simulink model "tx2"  (R2022a)
settings: Solver=FixedStepDiscrete  StartTime=0.0  StopTime=3.1e6  FixedStep=1  RelTol=1e-3
undefined symbols (not defined in the file or in its folder): rom_bf1, rom_bf2, rom_bf3, rom_bf4, rom_bf5, rom_bf6, rom_bf7, rom_bf8, rom_pilot_tt
libraries: hdlsllib x809, whdlutilities x460, whdlmod x104, whdledac x26, simulink x3
(part 1 of 27)
settings Model: SimulationMode=accelerator  Creator=admin  LastModifiedBy=admin
settings DataIOCC: ExternalInput=data_tt,valid_tt  LoadExternalInput=on

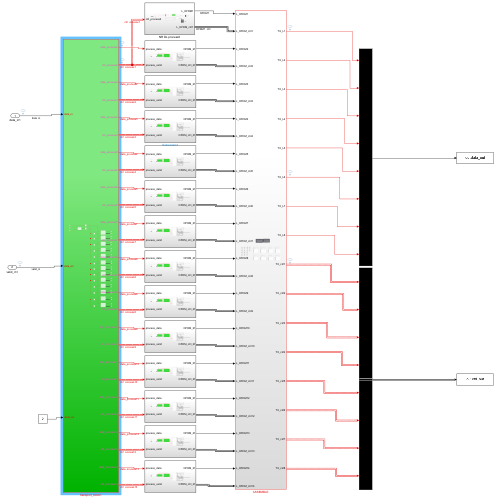
[thumbnail: Simulink's stored preview of the top-level diagram]
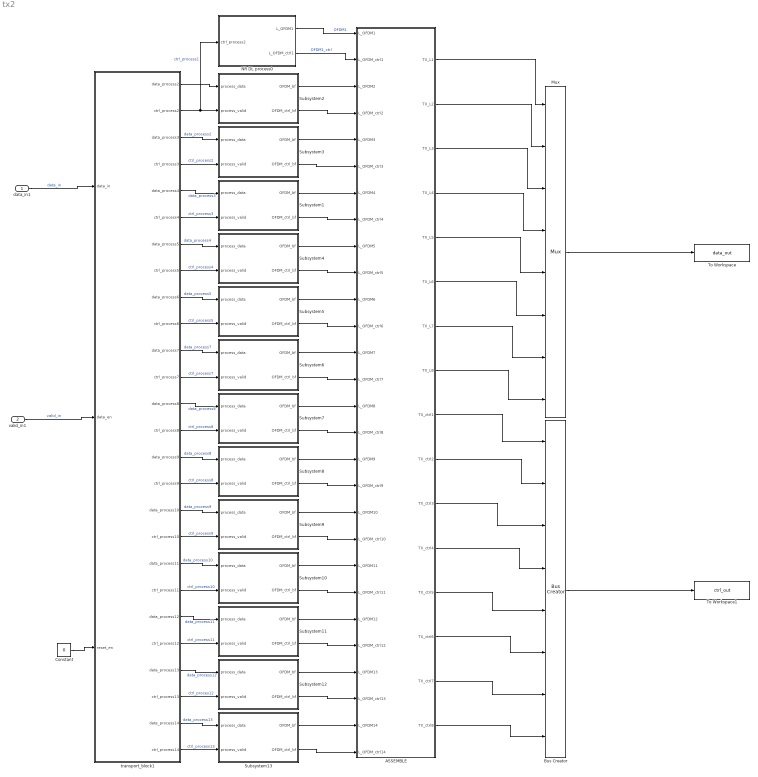
== system tx2 ==
  data_in1 : Inport  OutDataTypeStr=boolean
  valid_in1 : Inport  Port=2  OutDataTypeStr=boolean
  ASSEMBLE : Subsystem
  Bus Creator : BusCreator  Inputs=8
  Constant : Constant  Value=0  OutDataTypeStr=boolean
  Mux : Mux  Inputs=8
  NR DL process0 : Subsystem
  Subsystem1 : Subsystem
  Subsystem10 : Subsystem
  Subsystem11 : Subsystem
  Subsystem12 : Subsystem
  Subsystem13 : Subsystem
  Subsystem2 : Subsystem
  Subsystem3 : Subsystem
  Subsystem4 : Subsystem
  Subsystem5 : Subsystem
  Subsystem6 : Subsystem
  Subsystem7 : Subsystem
  Subsystem8 : Subsystem
  Subsystem9 : Subsystem
  To Workspace : ToWorkspace  VariableName=data_out  SaveFormat=Timeseries  SampleTime=-1
  To Workspace1 : ToWorkspace  VariableName=ctrl_out  SaveFormat=Timeseries  SampleTime=-1
  transport_block1 : Subsystem
  wires:
  ASSEMBLE/5(TX_L5) -> Mux/5
  transport_block1/22(ctrl_process12) -> Subsystem11/2(process_valid)  "ctrl_process11"
  Subsystem10/2(OFDM_ctrl_bf) -> ASSEMBLE/22(L_OFDM_ctrl11)
  ASSEMBLE/9(TX_ctrl1) -> Bus Creator/1
  transport_block1/25(data_process14) -> Subsystem13/1(process_data)  "data_process13"
  Subsystem11/2(OFDM_ctrl_bf) -> ASSEMBLE/24(L_OFDM_ctrl12)
  Subsystem10/1(OFDM_bf) -> ASSEMBLE/21(L_OFDM11)
  Subsystem12/2(OFDM_ctrl_bf) -> ASSEMBLE/26(L_OFDM_ctrl13)
  Subsystem9/2(OFDM_ctrl_bf) -> ASSEMBLE/20(L_OFDM_ctrl10)
  transport_block1/17(data_process10) -> Subsystem9/1(process_data)  "data_process9"
  transport_block1/20(ctrl_process11) -> Subsystem10/2(process_valid)  "ctrl_process10"
  transport_block1/8(ctrl_process5) -> Subsystem4/2(process_valid)  "ctrl_process4"
  Subsystem12/1(OFDM_bf) -> ASSEMBLE/25(L_OFDM13)
  transport_block1/14(ctrl_process8) -> Subsystem7/2(process_valid)  "ctrl_process8"
  Subsystem8/2(OFDM_ctrl_bf) -> ASSEMBLE/18(L_OFDM_ctrl9)
  Subsystem8/1(OFDM_bf) -> ASSEMBLE/17(L_OFDM9)
  transport_block1/16(ctrl_process9) -> Subsystem8/2(process_valid)  "ctrl_process8"
  Subsystem1/1(OFDM_bf) -> ASSEMBLE/7(L_OFDM4)
  Subsystem3/2(OFDM_ctrl_bf) -> ASSEMBLE/6(L_OFDM_ctrl3)
  transport_block1/4(ctrl_process3) -> Subsystem3/2(process_valid)  "ctrl_process2"
  Subsystem7/1(OFDM_bf) -> ASSEMBLE/15(L_OFDM8)
  Subsystem6/2(OFDM_ctrl_bf) -> ASSEMBLE/14(L_OFDM_ctrl7)
  transport_block1/13(data_process8) -> Subsystem7/1(process_data)  "data_process8"
  Subsystem2/2(OFDM_ctrl_bf) -> ASSEMBLE/4(L_OFDM_ctrl2)
  transport_block1/9(data_process6) -> Subsystem5/1(process_data)  "data_process5"
  transport_block1/12(ctrl_process7) -> Subsystem6/2(process_valid)  "ctrl_process7"
  Subsystem2/1(OFDM_bf) -> ASSEMBLE/3(L_OFDM2)
  Subsystem3/1(OFDM_bf) -> ASSEMBLE/5(L_OFDM3)
  ASSEMBLE/2(TX_L2) -> Mux/2
  Subsystem13/1(OFDM_bf) -> ASSEMBLE/27(L_OFDM14)
  transport_block1/10(ctrl_process6) -> Subsystem5/2(process_valid)  "ctrl_process5"
  transport_block1/6(ctrl_process4) -> Subsystem1/2(process_valid)  "ctrl_process3"
  Subsystem4/1(OFDM_bf) -> ASSEMBLE/9(L_OFDM5)
  Subsystem9/1(OFDM_bf) -> ASSEMBLE/19(L_OFDM10)
  Subsystem6/1(OFDM_bf) -> ASSEMBLE/13(L_OFDM7)
  Subsystem1/2(OFDM_ctrl_bf) -> ASSEMBLE/8(L_OFDM_ctrl4)
  transport_block1/18(ctrl_process10) -> Subsystem9/2(process_valid)  "ctrl_process9"
  ASSEMBLE/15(TX_ctrl7) -> Bus Creator/7
  Constant/1 -> transport_block1/3(reset_en)
  transport_block1/21(data_process12) -> Subsystem11/1(process_data)  "data_process11"
  transport_block1/24(ctrl_process13) -> Subsystem12/2(process_valid)  "ctrl_proces12"
  transport_block1/23(data_process13) -> Subsystem12/1(process_data)  "data_process12"
  ASSEMBLE/10(TX_ctrl2) -> Bus Creator/2
  Subsystem11/1(OFDM_bf) -> ASSEMBLE/23(L_OFDM12)
  valid_in1/1 -> transport_block1/2(data_en)  "valid_in"
  Subsystem4/2(OFDM_ctrl_bf) -> ASSEMBLE/10(L_OFDM_ctrl5)
  ASSEMBLE/1(TX_L1) -> Mux/1
  ASSEMBLE/4(TX_L4) -> Mux/4
  ASSEMBLE/12(TX_ctrl4) -> Bus Creator/4
  transport_block1/5(data_process4) -> Subsystem1/1(process_data)  "data_process3"
  NR DL process0/2(L_OFDM_ctrl1) -> ASSEMBLE/2(L_OFDM_ctrl1)  "OFDM1_ctrl"
  transport_block1/15(data_process9) -> Subsystem8/1(process_data)  "data_process8"
  ASSEMBLE/3(TX_L3) -> Mux/3
  ASSEMBLE/6(TX_L6) -> Mux/6
  ASSEMBLE/14(TX_ctrl6) -> Bus Creator/6
  ASSEMBLE/16(TX_ctrl8) -> Bus Creator/8
  transport_block1/11(data_process7) -> Subsystem6/1(process_data)  "data_process7"
  ASSEMBLE/7(TX_L7) -> Mux/7
  transport_block1/3(data_process3) -> Subsystem3/1(process_data)  "data_process2"
  NR DL process0/1(L_OFDM1) -> ASSEMBLE/1(L_OFDM1)  "OFDM1"
  transport_block1/26(ctrl_process14) -> Subsystem13/2(process_valid)  "ctrl_process13"
  ASSEMBLE/11(TX_ctrl3) -> Bus Creator/3
  data_in1/1 -> transport_block1/1(data_in)  "data_in"
  Subsystem5/2(OFDM_ctrl_bf) -> ASSEMBLE/12(L_OFDM_ctrl6)
  Subsystem7/2(OFDM_ctrl_bf) -> ASSEMBLE/16(L_OFDM_ctrl8)
  transport_block1/2(ctrl_process2) -> Subsystem2/2(process_valid), NR DL process0/1(ctrl_process2)  "ctrl_process1"
  transport_block1/19(data_process11) -> Subsystem10/1(process_data)  "data_process10"
  transport_block1/1(data_process2) -> Subsystem2/1(process_data)
  ASSEMBLE/8(TX_L8) -> Mux/8
  Subsystem5/1(OFDM_bf) -> ASSEMBLE/11(L_OFDM6)
  Subsystem13/2(OFDM_ctrl_bf) -> ASSEMBLE/28(L_OFDM_ctrl14)
  ASSEMBLE/13(TX_ctrl5) -> Bus Creator/5
  transport_block1/7(data_process5) -> Subsystem4/1(process_data)  "data_process4"
  Bus Creator/1 -> To Workspace1/1
  Mux/1 -> To Workspace/1

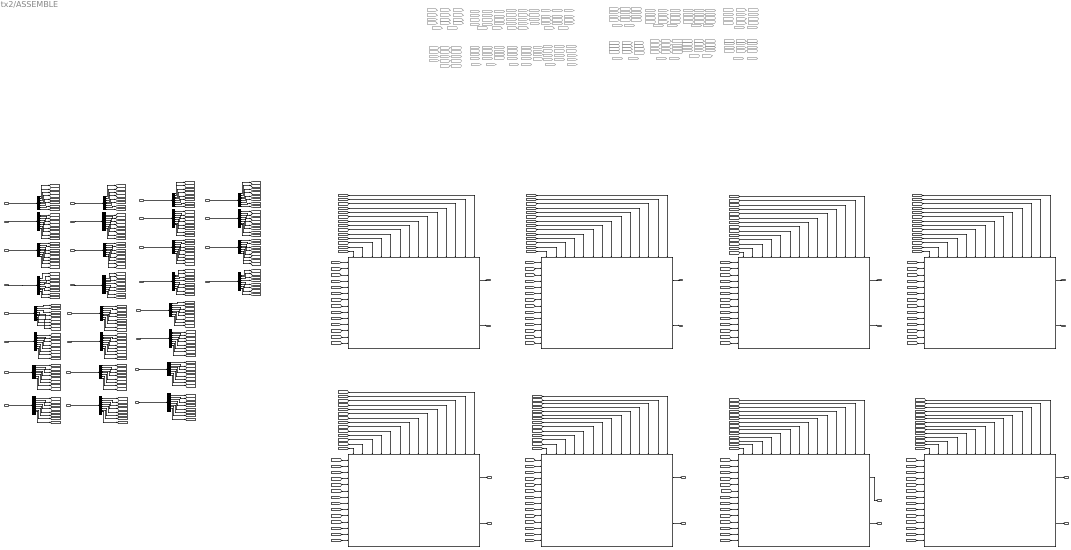
== system tx2/ASSEMBLE ==
  L_OFDM1 : Inport  PortDimensions=8
  L_OFDM_ctrl1 : Inport  Port=2  OutDataTypeStr=Bus: BUSOFDM1
  L_OFDM2 : Inport  Port=3  PortDimensions=8
  L_OFDM_ctrl2 : Inport  Port=4  OutDataTypeStr=Bus: BUSOFDM2
  L_OFDM3 : Inport  Port=5  PortDimensions=8
  L_OFDM_ctrl3 : Inport  Port=6  OutDataTypeStr=Bus: BUSOFDM3
  L_OFDM4 : Inport  Port=7  PortDimensions=8
  L_OFDM_ctrl4 : Inport  Port=8  OutDataTypeStr=Bus: BUSOFDM4
  L_OFDM5 : Inport  Port=9  PortDimensions=8
  L_OFDM_ctrl5 : Inport  Port=10  OutDataTypeStr=Bus: BUSOFDM5
  L_OFDM6 : Inport  Port=11  PortDimensions=8
  L_OFDM_ctrl6 : Inport  Port=12  OutDataTypeStr=Bus: BUSOFDM6
  L_OFDM7 : Inport  Port=13  PortDimensions=8
  L_OFDM_ctrl7 : Inport  Port=14  OutDataTypeStr=Bus: BUSOFDM7
  L_OFDM8 : Inport  Port=15  PortDimensions=8
  L_OFDM_ctrl8 : Inport  Port=16  OutDataTypeStr=Bus: BUSOFDM8
  L_OFDM9 : Inport  Port=17  PortDimensions=8
  L_OFDM_ctrl9 : Inport  Port=18  OutDataTypeStr=Bus: BUSOFDM9
  L_OFDM10 : Inport  Port=19  PortDimensions=8
  L_OFDM_ctrl10 : Inport  Port=20  OutDataTypeStr=Bus: BUSOFDM10
  L_OFDM11 : Inport  Port=21  PortDimensions=8
  L_OFDM_ctrl11 : Inport  Port=22  OutDataTypeStr=Bus: BUSOFDM11
  L_OFDM12 : Inport  Port=23  PortDimensions=8
  L_OFDM_ctrl12 : Inport  Port=24  OutDataTypeStr=Bus: BUSOFDM12
  L_OFDM13 : Inport  Port=25  PortDimensions=8
  L_OFDM_ctrl13 : Inport  Port=26  OutDataTypeStr=Bus: BUSOFDM13
  L_OFDM14 : Inport  Port=27  PortDimensions=8
  L_OFDM_ctrl14 : Inport  Port=28  OutDataTypeStr=Bus: BUSOFDM14
  Bus Selector{,2..13} (13 alike) : BusSelector  OutputSignals=L1,L2,L3,L4,L5,L6,L7,L8
  Bus Selector1 : BusSelector  OutputSignals=rom_valid (signal 1),rom_valid (signal 2),rom_valid (signal 3),rom_valid (signal 4),rom_valid (signal 5),rom_valid (signal 6),rom_valid (signal 7),rom_valid (signal 8)
  Demux{,2,4,6,8,10,12,14,16,18,24,26,28,30} (14 alike) : Demux  Outputs=8
  From : From  Commented=on  GotoTag=OFDM1_L1
  From1 : From  Commented=on  GotoTag=OFDM1_L2
  From10 : From  Commented=on  GotoTag=OFDM1_L3_C
  From100 : From  Commented=on  GotoTag=OFDM7_L5
  From101 : From  Commented=on  GotoTag=OFDM7_L6
  From102 : From  Commented=on  GotoTag=OFDM7_L7
  From103 : From  Commented=on  GotoTag=OFDM7_L8
  From104 : From  Commented=on  GotoTag=OFDM7_L1_C
  From105 : From  Commented=on  GotoTag=OFDM7_L2_C
  From106 : From  Commented=on  GotoTag=OFDM7_L3_C
  From107 : From  Commented=on  GotoTag=OFDM7_L4_C
  From108 : From  Commented=on  GotoTag=OFDM7_L5_C
  From109 : From  Commented=on  GotoTag=OFDM7_L6_C
  From11 : From  Commented=on  GotoTag=OFDM1_L4_C
  From110 : From  Commented=on  GotoTag=OFDM7_L7_C
  From111 : From  Commented=on  GotoTag=OFDM7_L8_C
  From112 : From  Commented=on  GotoTag=OFDM8_L1
  From113 : From  Commented=on  GotoTag=OFDM8_L2
  From114 : From  Commented=on  GotoTag=OFDM8_L3
  From115 : From  Commented=on  GotoTag=OFDM8_L4
  From116 : From  Commented=on  GotoTag=OFDM8_L5
  From117 : From  Commented=on  GotoTag=OFDM8_L6
  From118 : From  Commented=on  GotoTag=OFDM8_L7
  From119 : From  Commented=on  GotoTag=OFDM8_L8
  From12 : From  Commented=on  GotoTag=OFDM1_L5_C
  From120 : From  Commented=on  GotoTag=OFDM8_L1_C
  From121 : From  Commented=on  GotoTag=OFDM8_L2_C
  From122 : From  Commented=on  GotoTag=OFDM8_L3_C
  From123 : From  Commented=on  GotoTag=OFDM8_L4_C
  From124 : From  Commented=on  GotoTag=OFDM8_L5_C
  From125 : From  Commented=on  GotoTag=OFDM8_L6_C
  From126 : From  Commented=on  GotoTag=OFDM8_L7_C
  From127 : From  Commented=on  GotoTag=OFDM8_L8_C
  From128 : From  Commented=on  GotoTag=OFDM9_L1
  From129 : From  Commented=on  GotoTag=OFDM9_L2
  From13 : From  Commented=on  GotoTag=OFDM1_L6_C
  From130 : From  Commented=on  GotoTag=OFDM9_L3
  From131 : From  Commented=on  GotoTag=OFDM9_L4
  From132 : From  Commented=on  GotoTag=OFDM9_L5
  From133 : From  Commented=on  GotoTag=OFDM9_L6
  From134 : From  Commented=on  GotoTag=OFDM9_L7
  From135 : From  Commented=on  GotoTag=OFDM9_L8
  From136 : From  Commented=on  GotoTag=OFDM9_L1_C
  From137 : From  Commented=on  GotoTag=OFDM9_L2_C
  From138 : From  Commented=on  GotoTag=OFDM9_L3_C
  From139 : From  Commented=on  GotoTag=OFDM9_L4_C
  From14 : From  Commented=on  GotoTag=OFDM1_L7_C
  From140 : From  Commented=on  GotoTag=OFDM9_L5_C
  From141 : From  Commented=on  GotoTag=OFDM9_L7_C
  From142 : From  Commented=on  GotoTag=OFDM9_L6_C
  From143 : From  Commented=on  GotoTag=OFDM9_L8_C
  From144 : From  Commented=on  GotoTag=OFDM10_L1
  From145 : From  Commented=on  GotoTag=OFDM10_L2
  From146 : From  Commented=on  GotoTag=OFDM10_L3
  From147 : From  Commented=on  GotoTag=OFDM10_L4
  From148 : From  Commented=on  GotoTag=OFDM10_L5
  From149 : From  Commented=on  GotoTag=OFDM10_L6
  From15 : From  Commented=on  GotoTag=OFDM1_L8_C
  From150 : From  Commented=on  GotoTag=OFDM10_L7
  From151 : From  Commented=on  GotoTag=OFDM10_L8
  From152 : From  Commented=on  GotoTag=OFDM10_L1_C
  From153 : From  Commented=on  GotoTag=OFDM10_L2_C
  From154 : From  Commented=on  GotoTag=OFDM10_L3_C
  From155 : From  Commented=on  GotoTag=OFDM10_L4_C
  From156 : From  Commented=on  GotoTag=OFDM10_L5_C
  From157 : From  Commented=on  GotoTag=OFDM10_L6_C
  From158 : From  Commented=on  GotoTag=OFDM10_L7_C
  From159 : From  Commented=on  GotoTag=OFDM10_L8_C
  From16 : From  Commented=on  GotoTag=OFDM2_L1
  From160 : From  Commented=on  GotoTag=OFDM11_L1
  From161 : From  Commented=on  GotoTag=OFDM11_L2
  From162 : From  Commented=on  GotoTag=OFDM11_L3
  From163 : From  Commented=on  GotoTag=OFDM11_L4
  From164 : From  Commented=on  GotoTag=OFDM11_L5
  From165 : From  Commented=on  GotoTag=OFDM11_L6
  From166 : From  Commented=on  GotoTag=OFDM11_L7
  From167 : From  Commented=on  GotoTag=OFDM11_L8
  From168 : From  Commented=on  GotoTag=OFDM11_L1_C
  From169 : From  Commented=on  GotoTag=OFDM11_L2_C
  From17 : From  Commented=on  GotoTag=OFDM2_L2
  From170 : From  Commented=on  GotoTag=OFDM11_L3_C
  From171 : From  Commented=on  GotoTag=OFDM11_L4_C
  From172 : From  Commented=on  GotoTag=OFDM11_L5_C
  From173 : From  Commented=on  GotoTag=OFDM11_L6_C
  From174 : From  Commented=on  GotoTag=OFDM11_L7_C
  From175 : From  Commented=on  GotoTag=OFDM11_L8_C
  From176 : From  Commented=on  GotoTag=OFDM12_L1
  From177 : From  Commented=on  GotoTag=OFDM12_L2
  From178 : From  Commented=on  GotoTag=OFDM12_L3
  From179 : From  Commented=on  GotoTag=OFDM12_L4
  From18 : From  Commented=on  GotoTag=OFDM2_L3
  From180 : From  Commented=on  GotoTag=OFDM12_L5
  From181 : From  Commented=on  GotoTag=OFDM12_L6
  From182 : From  Commented=on  GotoTag=OFDM12_L7
  From183 : From  Commented=on  GotoTag=OFDM12_L8
  From184 : From  Commented=on  GotoTag=OFDM12_L1_C
  From185 : From  Commented=on  GotoTag=OFDM12_L2_C
  From186 : From  Commented=on  GotoTag=OFDM12_L3_C
  From187 : From  Commented=on  GotoTag=OFDM12_L4_C
  From188 : From  Commented=on  GotoTag=OFDM12_L5_C
  From189 : From  Commented=on  GotoTag=OFDM12_L6_C
  From19 : From  Commented=on  GotoTag=OFDM2_L4
  From190 : From  Commented=on  GotoTag=OFDM12_L7_C
  From191 : From  Commented=on  GotoTag=OFDM12_L8_C
  From192 : From  Commented=on  GotoTag=OFDM13_L1
  From193 : From  Commented=on  GotoTag=OFDM13_L2
  From194 : From  Commented=on  GotoTag=OFDM13_L3
  From195 : From  Commented=on  GotoTag=OFDM13_L4
  From196 : From  Commented=on  GotoTag=OFDM13_L5
  From197 : From  Commented=on  GotoTag=OFDM13_L6
  From198 : From  Commented=on  GotoTag=OFDM13_L7
  From199 : From  Commented=on  GotoTag=OFDM13_L8
  From2 : From  Commented=on  GotoTag=OFDM1_L3
  From20 : From  Commented=on  GotoTag=OFDM2_L5
  From200 : From  Commented=on  GotoTag=OFDM13_L1_C
  From201 : From  Commented=on  GotoTag=OFDM13_L2_C
  From202 : From  Commented=on  GotoTag=OFDM13_L3_C
  From203 : From  Commented=on  GotoTag=OFDM13_L4_C
  From204 : From  Commented=on  GotoTag=OFDM13_L5_C
  From205 : From  Commented=on  GotoTag=OFDM13_L6_C
  From206 : From  Commented=on  GotoTag=OFDM13_L7_C
  From207 : From  Commented=on  GotoTag=OFDM13_L8_C
  From208 : From  Commented=on  GotoTag=OFDM14_L1
  From209 : From  Commented=on  GotoTag=OFDM14_L2
  From21 : From  Commented=on  GotoTag=OFDM2_L6
  From210 : From  Commented=on  GotoTag=OFDM14_L3
  From211 : From  Commented=on  GotoTag=OFDM14_L4
  From212 : From  Commented=on  GotoTag=OFDM14_L5
  From213 : From  Commented=on  GotoTag=OFDM14_L6
  From214 : From  Commented=on  GotoTag=OFDM14_L7
  From215 : From  Commented=on  GotoTag=OFDM14_L8
  From216 : From  Commented=on  GotoTag=OFDM14_L1_C
  From217 : From  Commented=on  GotoTag=OFDM14_L2_C
  From218 : From  Commented=on  GotoTag=OFDM14_L3_C
  From219 : From  Commented=on  GotoTag=OFDM14_L4_C
  From22 : From  Commented=on  GotoTag=OFDM2_L7
  From220 : From  Commented=on  GotoTag=OFDM14_L5_C
  From221 : From  Commented=on  GotoTag=OFDM14_L6_C
  From222 : From  Commented=on  GotoTag=OFDM14_L7_C
  From223 : From  Commented=on  GotoTag=OFDM14_L8_C
  From23 : From  Commented=on  GotoTag=OFDM2_L8
  From24 : From  Commented=on  GotoTag=OFDM2_L1_C
  From25 : From  Commented=on  GotoTag=OFDM2_L2_C
  From26 : From  Commented=on  GotoTag=OFDM2_L3_C
  From27 : From  Commented=on  GotoTag=OFDM2_L4_C
  From28 : From  Commented=on  GotoTag=OFDM2_L5_C
  From29 : From  Commented=on  GotoTag=OFDM2_L6_C
  From3 : From  Commented=on  GotoTag=OFDM1_L4
  From30 : From  Commented=on  GotoTag=OFDM2_L7_C
  From31 : From  Commented=on  GotoTag=OFDM2_L8_C
  From32 : From  Commented=on  GotoTag=OFDM3_L1
  From33 : From  Commented=on  GotoTag=OFDM3_L2
  From34 : From  Commented=on  GotoTag=OFDM3_L3
  From35 : From  Commented=on  GotoTag=OFDM3_L4
  From36 : From  Commented=on  GotoTag=OFDM3_L5
  From37 : From  Commented=on  GotoTag=OFDM3_L6
  From38 : From  Commented=on  GotoTag=OFDM3_L7
  From39 : From  Commented=on  GotoTag=OFDM3_L8
  From4 : From  Commented=on  GotoTag=OFDM1_L5
  From40 : From  Commented=on  GotoTag=OFDM3_L1_C
  From41 : From  Commented=on  GotoTag=OFDM3_L2_C
  From42 : From  Commented=on  GotoTag=OFDM3_L3_C
  From43 : From  Commented=on  GotoTag=OFDM3_L4_C
  From44 : From  Commented=on  GotoTag=OFDM3_L5_C
  From45 : From  Commented=on  GotoTag=OFDM3_L6_C
  From46 : From  Commented=on  GotoTag=OFDM3_L7_C
  From47 : From  Commented=on  GotoTag=OFDM3_L8_C
  From48 : From  Commented=on  GotoTag=OFDM4_L1
  From49 : From  Commented=on  GotoTag=OFDM4_L2
  From5 : From  Commented=on  GotoTag=OFDM1_L6
  From50 : From  Commented=on  GotoTag=OFDM4_L3
  From51 : From  Commented=on  GotoTag=OFDM4_L4
  From52 : From  Commented=on  GotoTag=OFDM4_L5
  From53 : From  Commented=on  GotoTag=OFDM4_L6
  From54 : From  Commented=on  GotoTag=OFDM4_L7
  From55 : From  Commented=on  GotoTag=OFDM4_L8
  From56 : From  Commented=on  GotoTag=OFDM4_L1_C
  From57 : From  Commented=on  GotoTag=OFDM4_L2_C
  From58 : From  Commented=on  GotoTag=OFDM4_L3_C
  From59 : From  Commented=on  GotoTag=OFDM4_L4_C
  From6 : From  Commented=on  GotoTag=OFDM1_L7
  From60 : From  Commented=on  GotoTag=OFDM4_L5_C
  From61 : From  Commented=on  GotoTag=OFDM4_L6_C
  From62 : From  Commented=on  GotoTag=OFDM4_L7_C
  From63 : From  Commented=on  GotoTag=OFDM4_L8_C
  From64 : From  Commented=on  GotoTag=OFDM5_L1
  From65 : From  Commented=on  GotoTag=OFDM5_L2
  From66 : From  Commented=on  GotoTag=OFDM5_L3
  From67 : From  Commented=on  GotoTag=OFDM5_L4
  From68 : From  Commented=on  GotoTag=OFDM5_L5
  From69 : From  Commented=on  GotoTag=OFDM5_L6
  From7 : From  Commented=on  GotoTag=OFDM1_L8
  From70 : From  Commented=on  GotoTag=OFDM5_L7
  From71 : From  Commented=on  GotoTag=OFDM5_L8
  From72 : From  Commented=on  GotoTag=OFDM5_L1_C
  From73 : From  Commented=on  GotoTag=OFDM5_L2_C
  From74 : From  Commented=on  GotoTag=OFDM5_L3_C
  From75 : From  Commented=on  GotoTag=OFDM5_L4_C
  From76 : From  Commented=on  GotoTag=OFDM5_L5_C
  From77 : From  Commented=on  GotoTag=OFDM5_L6_C
  From78 : From  Commented=on  GotoTag=OFDM5_L7_C
  From79 : From  Commented=on  GotoTag=OFDM5_L8_C
  From8 : From  Commented=on  GotoTag=OFDM1_L1_C
  From80 : From  Commented=on  GotoTag=OFDM6_L1
  From81 : From  Commented=on  GotoTag=OFDM6_L2
  From82 : From  Commented=on  GotoTag=OFDM6_L3
  From83 : From  Commented=on  GotoTag=OFDM6_L4
  From84 : From  Commented=on  GotoTag=OFDM6_L5
  From85 : From  Commented=on  GotoTag=OFDM6_L6
  From86 : From  Commented=on  GotoTag=OFDM6_L7
  From87 : From  Commented=on  GotoTag=OFDM6_L8
  From88 : From  Commented=on  GotoTag=OFDM6_L1_C
  From89 : From  Commented=on  GotoTag=OFDM6_L2_C
  From9 : From  Commented=on  GotoTag=OFDM1_L2_C
  From90 : From  Commented=on  GotoTag=OFDM6_L3_C
  From91 : From  Commented=on  GotoTag=OFDM6_L4_C
  From92 : From  Commented=on  GotoTag=OFDM6_L5_C
  From93 : From  Commented=on  GotoTag=OFDM6_L6_C
  From94 : From  Commented=on  GotoTag=OFDM6_L7_C
  From95 : From  Commented=on  GotoTag=OFDM6_L8_C
  From96 : From  Commented=on  GotoTag=OFDM7_L1
  From97 : From  Commented=on  GotoTag=OFDM7_L2
  From98 : From  Commented=on  GotoTag=OFDM7_L3
  From99 : From  Commented=on  GotoTag=OFDM7_L4
  LAY1 : Subsystem
      settings: PortSchema="{\"entries\":[{\"content\":{\"sides\":[{\"content\":{\"connectorIds\":[\"In1\",\"In2\",\"In3\",\"In4\",\"In5\",\"In6\",\"In7\",\"In8\",\"In9\",\"In10\",\"In11\",\"In12\",\"In13\",\"In14\"]},\"type\":\"ConnectorPlacement.EquallySpacedRectSide\",\"uuid\":\"490598a8-c3f5-4389-b0d6-cf6a9e30693d\"},{\"content\":{\"connectorIds\":[\"Out1\",\"Out2\"],\"side\":\"RIGHT\"},\"type\":\"ConnectorPlacement.EquallySpacedRectSide\",\"uuid\":\"6437ac82-c6ba-4d32-8bfc-bd63e74c8be4\"},{\"content\":{\"connectorIds\":[\"In15\",\"In16\",\"In17\",\"In18\",\"In19\",\"In20\",\"In21\",\"In22\",\"In23\",\"In24\",\"In25\",\"In26\",\"In27\",\"In28\"],\"side\":\"TOP\"},\"type\":\"ConnectorPlacement.EquallySpacedRectSide\",\"uuid\":\"6de7b101-133c-4248-a10a-e7ae53670d39\"}]},\"type\":\"ConnectorPlacement.EquallySpacedConnector\",\"uuid\":\"6f2047fb-9444-475d-b0d6-20b25d9f763e\"}],\"packageUris\":[\"http://schema.mathworks.com/mf0/Connector/R2020b\"],\"version\":\"1.0\"}"
  LAY2 : Subsystem
      settings: PortSchema="{\"entries\":[{\"content\":{\"sides\":[{\"content\":{\"connectorIds\":[\"In1\",\"In2\",\"In3\",\"In4\",\"In5\",\"In6\",\"In7\",\"In8\",\"In9\",\"In10\",\"In11\",\"In12\",\"In13\",\"In14\"]},\"type\":\"ConnectorPlacement.EquallySpacedRectSide\",\"uuid\":\"490598a8-c3f5-4389-b0d6-cf6a9e30693d\"},{\"content\":{\"connectorIds\":[\"Out1\",\"Out2\"],\"side\":\"RIGHT\"},\"type\":\"ConnectorPlacement.EquallySpacedRectSide\",\"uuid\":\"6437ac82-c6ba-4d32-8bfc-bd63e74c8be4\"},{\"content\":{\"connectorIds\":[\"In15\",\"In16\",\"In17\",\"In18\",\"In19\",\"In20\",\"In21\",\"In22\",\"In23\",\"In24\",\"In25\",\"In26\",\"In27\",\"In28\"],\"side\":\"TOP\"},\"type\":\"ConnectorPlacement.EquallySpacedRectSide\",\"uuid\":\"6de7b101-133c-4248-a10a-e7ae53670d39\"}]},\"type\":\"ConnectorPlacement.EquallySpacedConnector\",\"uuid\":\"6f2047fb-9444-475d-b0d6-20b25d9f763e\"}],\"packageUris\":[\"http://schema.mathworks.com/mf0/Connector/R2020b\"],\"version\":\"1.0\"}"
  LAY3 : Subsystem
      settings: PortSchema="{\"entries\":[{\"content\":{\"sides\":[{\"content\":{\"connectorIds\":[\"In1\",\"In2\",\"In3\",\"In4\",\"In5\",\"In6\",\"In7\",\"In8\",\"In9\",\"In10\",\"In11\",\"In12\",\"In13\",\"In14\"]},\"type\":\"ConnectorPlacement.EquallySpacedRectSide\",\"uuid\":\"490598a8-c3f5-4389-b0d6-cf6a9e30693d\"},{\"content\":{\"connectorIds\":[\"Out1\",\"Out2\"],\"side\":\"RIGHT\"},\"type\":\"ConnectorPlacement.EquallySpacedRectSide\",\"uuid\":\"6437ac82-c6ba-4d32-8bfc-bd63e74c8be4\"},{\"content\":{\"connectorIds\":[\"In15\",\"In16\",\"In17\",\"In18\",\"In19\",\"In20\",\"In21\",\"In22\",\"In23\",\"In24\",\"In25\",\"In26\",\"In27\",\"In28\"],\"side\":\"TOP\"},\"type\":\"ConnectorPlacement.EquallySpacedRectSide\",\"uuid\":\"6de7b101-133c-4248-a10a-e7ae53670d39\"}]},\"type\":\"ConnectorPlacement.EquallySpacedConnector\",\"uuid\":\"6f2047fb-9444-475d-b0d6-20b25d9f763e\"}],\"packageUris\":[\"http://schema.mathworks.com/mf0/Connector/R2020b\"],\"version\":\"1.0\"}"
  LAY4 : Subsystem
      settings: PortSchema="{\"entries\":[{\"content\":{\"sides\":[{\"content\":{\"connectorIds\":[\"In1\",\"In2\",\"In3\",\"In4\",\"In5\",\"In6\",\"In7\",\"In8\",\"In9\",\"In10\",\"In11\",\"In12\",\"In13\",\"In14\"]},\"type\":\"ConnectorPlacement.EquallySpacedRectSide\",\"uuid\":\"490598a8-c3f5-4389-b0d6-cf6a9e30693d\"},{\"content\":{\"connectorIds\":[\"Out1\",\"Out2\"],\"side\":\"RIGHT\"},\"type\":\"ConnectorPlacement.EquallySpacedRectSide\",\"uuid\":\"6437ac82-c6ba-4d32-8bfc-bd63e74c8be4\"},{\"content\":{\"connectorIds\":[\"In15\",\"In16\",\"In17\",\"In18\",\"In19\",\"In20\",\"In21\",\"In22\",\"In23\",\"In24\",\"In25\",\"In26\",\"In27\",\"In28\"],\"side\":\"TOP\"},\"type\":\"ConnectorPlacement.EquallySpacedRectSide\",\"uuid\":\"6de7b101-133c-4248-a10a-e7ae53670d39\"}]},\"type\":\"ConnectorPlacement.EquallySpacedConnector\",\"uuid\":\"6f2047fb-9444-475d-b0d6-20b25d9f763e\"}],\"packageUris\":[\"http://schema.mathworks.com/mf0/Connector/R2020b\"],\"version\":\"1.0\"}"
  LAY5 : Subsystem
      settings: PortSchema="{\"entries\":[{\"content\":{\"sides\":[{\"content\":{\"connectorIds\":[\"In1\",\"In2\",\"In3\",\"In4\",\"In5\",\"In6\",\"In7\",\"In8\",\"In9\",\"In10\",\"In11\",\"In12\",\"In13\",\"In14\"]},\"type\":\"ConnectorPlacement.EquallySpacedRectSide\",\"uuid\":\"490598a8-c3f5-4389-b0d6-cf6a9e30693d\"},{\"content\":{\"connectorIds\":[\"Out1\",\"Out2\"],\"side\":\"RIGHT\"},\"type\":\"ConnectorPlacement.EquallySpacedRectSide\",\"uuid\":\"6437ac82-c6ba-4d32-8bfc-bd63e74c8be4\"},{\"content\":{\"connectorIds\":[\"In15\",\"In16\",\"In17\",\"In18\",\"In19\",\"In20\",\"In21\",\"In22\",\"In23\",\"In24\",\"In25\",\"In26\",\"In27\",\"In28\"],\"side\":\"TOP\"},\"type\":\"ConnectorPlacement.EquallySpacedRectSide\",\"uuid\":\"6de7b101-133c-4248-a10a-e7ae53670d39\"}]},\"type\":\"ConnectorPlacement.EquallySpacedConnector\",\"uuid\":\"6f2047fb-9444-475d-b0d6-20b25d9f763e\"}],\"packageUris\":[\"http://schema.mathworks.com/mf0/Connector/R2020b\"],\"version\":\"1.0\"}"
  LAY6 : Subsystem
      settings: PortSchema="{\"entries\":[{\"content\":{\"sides\":[{\"content\":{\"connectorIds\":[\"In1\",\"In2\",\"In3\",\"In4\",\"In5\",\"In6\",\"In7\",\"In8\",\"In9\",\"In10\",\"In11\",\"In12\",\"In13\",\"In14\"]},\"type\":\"ConnectorPlacement.EquallySpacedRectSide\",\"uuid\":\"490598a8-c3f5-4389-b0d6-cf6a9e30693d\"},{\"content\":{\"connectorIds\":[\"Out1\",\"Out2\"],\"side\":\"RIGHT\"},\"type\":\"ConnectorPlacement.EquallySpacedRectSide\",\"uuid\":\"6437ac82-c6ba-4d32-8bfc-bd63e74c8be4\"},{\"content\":{\"connectorIds\":[\"In15\",\"In16\",\"In17\",\"In18\",\"In19\",\"In20\",\"In21\",\"In22\",\"In23\",\"In24\",\"In25\",\"In26\",\"In27\",\"In28\"],\"side\":\"TOP\"},\"type\":\"ConnectorPlacement.EquallySpacedRectSide\",\"uuid\":\"6de7b101-133c-4248-a10a-e7ae53670d39\"}]},\"type\":\"ConnectorPlacement.EquallySpacedConnector\",\"uuid\":\"6f2047fb-9444-475d-b0d6-20b25d9f763e\"}],\"packageUris\":[\"http://schema.mathworks.com/mf0/Connector/R2020b\"],\"version\":\"1.0\"}"
  LAY7 : Subsystem
      settings: PortSchema="{\"entries\":[{\"content\":{\"sides\":[{\"content\":{\"connectorIds\":[\"In1\",\"In2\",\"In3\",\"In4\",\"In5\",\"In6\",\"In7\",\"In8\",\"In9\",\"In10\",\"In11\",\"In12\",\"In13\",\"In14\"]},\"type\":\"ConnectorPlacement.EquallySpacedRectSide\",\"uuid\":\"490598a8-c3f5-4389-b0d6-cf6a9e30693d\"},{\"content\":{\"connectorIds\":[\"Out1\",\"Out2\"],\"side\":\"RIGHT\"},\"type\":\"ConnectorPlacement.EquallySpacedRectSide\",\"uuid\":\"6437ac82-c6ba-4d32-8bfc-bd63e74c8be4\"},{\"content\":{\"connectorIds\":[\"In15\",\"In16\",\"In17\",\"In18\",\"In19\",\"In20\",\"In21\",\"In22\",\"In23\",\"In24\",\"In25\",\"In26\",\"In27\",\"In28\"],\"side\":\"TOP\"},\"type\":\"ConnectorPlacement.EquallySpacedRectSide\",\"uuid\":\"6de7b101-133c-4248-a10a-e7ae53670d39\"}]},\"type\":\"ConnectorPlacement.EquallySpacedConnector\",\"uuid\":\"6f2047fb-9444-475d-b0d6-20b25d9f763e\"}],\"packageUris\":[\"http://schema.mathworks.com/mf0/Connector/R2020b\"],\"version\":\"1.0\"}"
  LAY9 : Subsystem
      settings: PortSchema="{\"entries\":[{\"content\":{\"sides\":[{\"content\":{\"connectorIds\":[\"In1\",\"In2\",\"In3\",\"In4\",\"In5\",\"In6\",\"In7\",\"In8\",\"In9\",\"In10\",\"In11\",\"In12\",\"In13\",\"In14\"]},\"type\":\"ConnectorPlacement.EquallySpacedRectSide\",\"uuid\":\"490598a8-c3f5-4389-b0d6-cf6a9e30693d\"},{\"content\":{\"connectorIds\":[\"Out1\",\"Out2\"],\"side\":\"RIGHT\"},\"type\":\"ConnectorPlacement.EquallySpacedRectSide\",\"uuid\":\"6437ac82-c6ba-4d32-8bfc-bd63e74c8be4\"},{\"content\":{\"connectorIds\":[\"In15\",\"In16\",\"In17\",\"In18\",\"In19\",\"In20\",\"In21\",\"In22\",\"In23\",\"In24\",\"In25\",\"In26\",\"In27\",\"In28\"],\"side\":\"TOP\"},\"type\":\"ConnectorPlacement.EquallySpacedRectSide\",\"uuid\":\"6de7b101-133c-4248-a10a-e7ae53670d39\"}]},\"type\":\"ConnectorPlacement.EquallySpacedConnector\",\"uuid\":\"6f2047fb-9444-475d-b0d6-20b25d9f763e\"}],\"packageUris\":[\"http://schema.mathworks.com/mf0/Connector/R2020b\"],\"version\":\"1.0\"}"
  TX_L1 : Outport
      settings: SignalType=complex
  TX_L2 : Outport  Port=2
      settings: SignalType=complex
  TX_L3 : Outport  Port=3
      settings: SignalType=complex
  TX_L4 : Outport  Port=4
      settings: SignalType=complex
  TX_L5 : Outport  Port=5
      settings: SignalType=complex
  TX_L6 : Outport  Port=6
      settings: SignalType=complex
  TX_L7 : Outport  Port=7
      settings: SignalType=complex
  TX_L8 : Outport  Port=8
      settings: SignalType=complex
  TX_ctrl1 : Outport  Port=9  OutDataTypeStr=Bus: samplecontrol
  TX_ctrl2 : Outport  Port=10  OutDataTypeStr=Bus: samplecontrol
  TX_ctrl3 : Outport  Port=11  OutDataTypeStr=Bus: samplecontrol
  TX_ctrl4 : Outport  Port=12  OutDataTypeStr=Bus: samplecontrol
  TX_ctrl5 : Outport  Port=13  OutDataTypeStr=Bus: samplecontrol
  TX_ctrl6 : Outport  Port=14  OutDataTypeStr=Bus: samplecontrol
  TX_ctrl7 : Outport  Port=15  OutDataTypeStr=Bus: samplecontrol
  TX_ctrl8 : Outport  Port=16  OutDataTypeStr=Bus: samplecontrol
  wires:
  L_OFDM1/1 -> Demux/1
  L_OFDM_ctrl1/1 -> Bus Selector1/1
  L_OFDM_ctrl2/1 -> Bus Selector/1
  L_OFDM2/1 -> Demux2/1
  L_OFDM4/1 -> Demux6/1
  L_OFDM_ctrl4/1 -> Bus Selector3/1
  L_OFDM_ctrl3/1 -> Bus Selector2/1
  L_OFDM3/1 -> Demux4/1
  Demux/1 -> [OFDM1_L1]  "OFDM1"
  Demux/2 -> [OFDM1_L2]
  Demux/3 -> [OFDM1_L3]
  Demux/4 -> [OFDM1_L4]
  Demux/5 -> [OFDM1_L5]
  Demux/6 -> [OFDM1_L6]
  Demux/7 -> [OFDM1_L7]
  Demux/8 -> [OFDM1_L8]
  Bus Selector1/1 -> [OFDM1_L1_C]  "<rom_valid (signal 1)>"
  Bus Selector1/2 -> [OFDM1_L2_C]  "<rom_valid (signal 2)>"
  Bus Selector1/3 -> [OFDM1_L3_C]  "<rom_valid (signal 3)>"
  Bus Selector1/4 -> [OFDM1_L4_C]  "<rom_valid (signal 4)>"
  Bus Selector1/5 -> [OFDM1_L5_C]  "<rom_valid (signal 5)>"
  Bus Selector1/6 -> [OFDM1_L6_C]  "<rom_valid (signal 6)>"
  Bus Selector1/7 -> [OFDM1_L7_C]  "<rom_valid (signal 7)>"
  Bus Selector1/8 -> [OFDM1_L8_C]  "<rom_valid (signal 8)>"
  Demux2/1 -> [OFDM2_L1]  "OFDM2"
  Demux2/2 -> [OFDM2_L2]
  Demux2/3 -> [OFDM2_L3]
  Demux2/4 -> [OFDM2_L4]
  Demux2/5 -> [OFDM2_L5]
  Demux2/6 -> [OFDM2_L6]
  Demux2/7 -> [OFDM2_L7]
  Demux2/8 -> [OFDM2_L8]
  Bus Selector/1 -> [OFDM2_L1_C]  "<L1>"
  Bus Selector/2 -> [OFDM2_L2_C]  "<L2>"
  Bus Selector/3 -> [OFDM2_L3_C]  "<L3>"
  Bus Selector/4 -> [OFDM2_L4_C]  "<L4>"
  Bus Selector/5 -> [OFDM2_L5_C]  "<L5>"
  Bus Selector/6 -> [OFDM2_L6_C]  "<L6>"
  Bus Selector/7 -> [OFDM2_L7_C]  "<L7>"
  Bus Selector/8 -> [OFDM2_L8_C]  "<L8>"
  Demux4/1 -> [OFDM3_L1]  "OFDM3"
  Demux4/2 -> [OFDM3_L2]
  Demux4/3 -> [OFDM3_L3]
  Demux4/4 -> [OFDM3_L4]
  Demux4/5 -> [OFDM3_L5]
  Demux4/6 -> [OFDM3_L6]
  Demux4/7 -> [OFDM3_L7]
  Demux4/8 -> [OFDM3_L8]
  Bus Selector2/1 -> [OFDM3_L1_C]  "<L1>"
  Bus Selector2/2 -> [OFDM3_L2_C]  "<L2>"
  Bus Selector2/3 -> [OFDM3_L3_C]  "<L3>"
  Bus Selector2/4 -> [OFDM3_L4_C]  "<L4>"
  Bus Selector2/5 -> [OFDM3_L5_C]  "<L5>"
  Bus Selector2/6 -> [OFDM3_L6_C]  "<L6>"
  Bus Selector2/7 -> [OFDM3_L7_C]  "<L7>"
  Bus Selector2/8 -> [OFDM3_L8_C]  "<L8>"
  Demux6/1 -> [OFDM4_L1]  "OFDM4"
  Demux6/2 -> [OFDM4_L2]
  Demux6/3 -> [OFDM4_L3]
  Demux6/4 -> [OFDM4_L4]
  Demux6/5 -> [OFDM4_L5]
  Demux6/6 -> [OFDM4_L6]
  Demux6/7 -> [OFDM4_L7]
  Demux6/8 -> [OFDM4_L8]
  Bus Selector3/1 -> [OFDM4_L1_C]  "<L1>"
  Bus Selector3/2 -> [OFDM4_L2_C]  "<L2>"
  Bus Selector3/3 -> [OFDM4_L3_C]  "<L3>"
  Bus Selector3/4 -> [OFDM4_L4_C]  "<L4>"
  Bus Selector3/5 -> [OFDM4_L5_C]  "<L5>"
  Bus Selector3/6 -> [OFDM4_L6_C]  "<L6>"
  Bus Selector3/7 -> [OFDM4_L7_C]  "<L7>"
  Bus Selector3/8 -> [OFDM4_L8_C]  "<L8>"
  Bus Selector4/8 -> [OFDM8_L8_C]  "<L8>"
  Bus Selector4/7 -> [OFDM8_L7_C]  "<L7>"
  Bus Selector4/6 -> [OFDM8_L6_C]  "<L6>"
  Bus Selector4/5 -> [OFDM8_L5_C]  "<L5>"
  Bus Selector4/4 -> [OFDM8_L4_C]  "<L4>"
  Bus Selector4/3 -> [OFDM8_L3_C]  "<L3>"
  Bus Selector4/2 -> [OFDM8_L2_C]  "<L2>"
  Bus Selector4/1 -> [OFDM8_L1_C]  "<L1>"
  Demux14/8 -> [OFDM8_L8]
  Demux14/7 -> [OFDM8_L7]
  Demux14/6 -> [OFDM8_L6]
  Demux14/5 -> [OFDM8_L5]
  Demux14/4 -> [OFDM8_L4]
  Demux14/3 -> [OFDM8_L3]
  Demux14/2 -> [OFDM8_L2]
  Demux14/1 -> [OFDM8_L1]  "OFDM8"
  Bus Selector5/8 -> [OFDM7_L8_C]  "<L8>"
  Bus Selector5/7 -> [OFDM7_L7_C]  "<L7>"
  Bus Selector5/6 -> [OFDM7_L6_C]  "<L6>"
  Bus Selector5/5 -> [OFDM7_L5_C]  "<L5>"
  Bus Selector5/4 -> [OFDM7_L4_C]  "<L4>"
  Bus Selector5/3 -> [OFDM7_L3_C]  "<L3>"
  Bus Selector5/2 -> [OFDM7_L2_C]  "<L2>"
  Bus Selector5/1 -> [OFDM7_L1_C]  "<L1>"
  Demux12/8 -> [OFDM7_L8]
  Demux12/7 -> [OFDM7_L7]
  Demux12/6 -> [OFDM7_L6]
  Demux12/5 -> [OFDM7_L5]
  Demux12/4 -> [OFDM7_L4]
  Demux12/3 -> [OFDM7_L3]
  Demux12/2 -> [OFDM7_L2]
  Demux12/1 -> [OFDM7_L1]  "OFDM7"
  Bus Selector6/8 -> [OFDM6_L8_C]  "<L8>"
  Bus Selector6/7 -> [OFDM6_L7_C]  "<L7>"
  Bus Selector6/6 -> [OFDM6_L6_C]  "<L6>"
  Bus Selector6/5 -> [OFDM6_L5_C]  "<L5>"
  Bus Selector6/4 -> [OFDM6_L4_C]  "<L4>"
  Bus Selector6/3 -> [OFDM6_L3_C]  "<L3>"
  Bus Selector6/2 -> [OFDM6_L2_C]  "<L2>"
  Bus Selector6/1 -> [OFDM6_L1_C]  "<L1>"
  Demux10/8 -> [OFDM6_L8]
  Demux10/7 -> [OFDM6_L7]
  Demux10/6 -> [OFDM6_L6]
  Demux10/5 -> [OFDM6_L5]
  Demux10/4 -> [OFDM6_L4]
  Demux10/3 -> [OFDM6_L3]
  Demux10/2 -> [OFDM6_L2]
  Demux10/1 -> [OFDM6_L1]  "OFDM6"
  Bus Selector7/8 -> [OFDM5_L8_C]  "<L8>"
  Bus Selector7/7 -> [OFDM5_L7_C]  "<L7>"
  Bus Selector7/6 -> [OFDM5_L6_C]  "<L6>"
  Bus Selector7/5 -> [OFDM5_L5_C]  "<L5>"
  Bus Selector7/4 -> [OFDM5_L4_C]  "<L4>"
  Bus Selector7/3 -> [OFDM5_L3_C]  "<L3>"
  Bus Selector7/2 -> [OFDM5_L2_C]  "<L2>"
  Bus Selector7/1 -> [OFDM5_L1_C]  "<L1>"
  Demux8/8 -> [OFDM5_L8]
  Demux8/7 -> [OFDM5_L7]
  Demux8/6 -> [OFDM5_L6]
  Demux8/5 -> [OFDM5_L5]
  Demux8/4 -> [OFDM5_L4]
  Demux8/3 -> [OFDM5_L3]
  Demux8/2 -> [OFDM5_L2]
  Demux8/1 -> [OFDM5_L1]  "OFDM5"
  L_OFDM7/1 -> Demux12/1
  L_OFDM_ctrl7/1 -> Bus Selector5/1
  L_OFDM_ctrl8/1 -> Bus Selector4/1
  L_OFDM8/1 -> Demux14/1
  L_OFDM6/1 -> Demux10/1
  L_OFDM_ctrl6/1 -> Bus Selector6/1
  L_OFDM_ctrl5/1 -> Bus Selector7/1
  L_OFDM5/1 -> Demux8/1
  L_OFDM13/1 -> Demux30/1
  L_OFDM_ctrl13/1 -> Bus Selector12/1
  L_OFDM_ctrl14/1 -> Bus Selector13/1
  L_OFDM14/1 -> Demux18/1
  Demux30/1 -> [OFDM13_L1]  "OFDM13"
  Demux30/2 -> [OFDM13_L2]
  Demux30/3 -> [OFDM13_L3]
  Demux30/4 -> [OFDM13_L4]
  Demux30/5 -> [OFDM13_L5]
  Demux30/6 -> [OFDM13_L6]
  Demux30/7 -> [OFDM13_L7]
  Demux30/8 -> [OFDM13_L8]
  Bus Selector12/1 -> [OFDM13_L1_C]  "<L1>"
  Bus Selector12/2 -> [OFDM13_L2_C]  "<L2>"
  Bus Selector12/3 -> [OFDM13_L3_C]  "<L3>"
  Bus Selector12/4 -> [OFDM13_L4_C]  "<L4>"
  Bus Selector12/5 -> [OFDM13_L5_C]  "<L5>"
  Bus Selector12/6 -> [OFDM13_L6_C]  "<L6>"
  Bus Selector12/7 -> [OFDM13_L7_C]  "<L7>"
  Bus Selector12/8 -> [OFDM13_L8_C]  "<L8>"
  Demux18/1 -> [OFDM14_L1]  "OFDM14"
  Demux18/2 -> [OFDM14_L2]
  Demux18/3 -> [OFDM14_L3]
  Demux18/4 -> [OFDM14_L4]
  Demux18/5 -> [OFDM14_L5]
  Demux18/6 -> [OFDM14_L6]
  Demux18/7 -> [OFDM14_L7]
  Demux18/8 -> [OFDM14_L8]
  Bus Selector13/1 -> [OFDM14_L1_C]  "<L1>"
  Bus Selector13/2 -> [OFDM14_L2_C]  "<L2>"
  Bus Selector13/3 -> [OFDM14_L3_C]  "<L3>"
  Bus Selector13/4 -> [OFDM14_L4_C]  "<L4>"
  Bus Selector13/5 -> [OFDM14_L5_C]  "<L5>"
  Bus Selector13/6 -> [OFDM14_L6_C]  "<L6>"
  Bus Selector13/7 -> [OFDM14_L7_C]  "<L7>"
  Bus Selector13/8 -> [OFDM14_L8_C]  "<L8>"
  Bus Selector11/8 -> [OFDM12_L8_C]  "<L8>"
  Bus Selector11/7 -> [OFDM12_L7_C]  "<L7>"
  Bus Selector11/6 -> [OFDM12_L6_C]  "<L6>"
  Bus Selector11/5 -> [OFDM12_L5_C]  "<L5>"
  Bus Selector11/4 -> [OFDM12_L4_C]  "<L4>"
  Bus Selector11/3 -> [OFDM12_L3_C]  "<L3>"
  Bus Selector11/2 -> [OFDM12_L2_C]  "<L2>"
  Bus Selector11/1 -> [OFDM12_L1_C]  "<L1>"
  Demux28/8 -> [OFDM12_L8]
  Demux28/7 -> [OFDM12_L7]
  Demux28/6 -> [OFDM12_L6]
  Demux28/5 -> [OFDM12_L5]
  Demux28/4 -> [OFDM12_L4]
  Demux28/3 -> [OFDM12_L3]
  Demux28/2 -> [OFDM12_L2]
  Demux28/1 -> [OFDM12_L1]  "OFDM12"
  Bus Selector10/8 -> [OFDM11_L8_C]  "<L8>"
  Bus Selector10/7 -> [OFDM11_L7_C]  "<L7>"
  Bus Selector10/6 -> [OFDM11_L6_C]  "<L6>"
  Bus Selector10/5 -> [OFDM11_L5_C]  "<L5>"
  Bus Selector10/4 -> [OFDM11_L4_C]  "<L4>"
  Bus Selector10/3 -> [OFDM11_L3_C]  "<L3>"
  Bus Selector10/2 -> [OFDM11_L2_C]  "<L2>"
  Bus Selector10/1 -> [OFDM11_L1_C]  "<L1>"
  Demux26/8 -> [OFDM11_L8]
  Demux26/7 -> [OFDM11_L7]
  Demux26/6 -> [OFDM11_L6]
  Demux26/5 -> [OFDM11_L5]
  Demux26/4 -> [OFDM11_L4]
  Demux26/3 -> [OFDM11_L3]
  Demux26/2 -> [OFDM11_L2]
  Demux26/1 -> [OFDM11_L1]  "OFDM11"
  Bus Selector9/8 -> [OFDM10_L8_C]  "<L8>"
  Bus Selector9/7 -> [OFDM10_L7_C]  "<L7>"
  Bus Selector9/6 -> [OFDM10_L6_C]  "<L6>"
  Bus Selector9/5 -> [OFDM10_L5_C]  "<L5>"
  Bus Selector9/4 -> [OFDM10_L4_C]  "<L4>"
  Bus Selector9/3 -> [OFDM10_L3_C]  "<L3>"
  Bus Selector9/2 -> [OFDM10_L2_C]  "<L2>"
  Bus Selector9/1 -> [OFDM10_L1_C]  "<L1>"
  Demux24/8 -> [OFDM10_L8]
  Demux24/7 -> [OFDM10_L7]
  Demux24/6 -> [OFDM10_L6]
  Demux24/5 -> [OFDM10_L5]
  Demux24/4 -> [OFDM10_L4]
  Demux24/3 -> [OFDM10_L3]
  Demux24/2 -> [OFDM10_L2]
  Demux24/1 -> [OFDM10_L1]  "OFDM10"
  Bus Selector8/8 -> [OFDM9_L8_C]  "<L8>"
  Bus Selector8/7 -> [OFDM9_L7_C]  "<L7>"
  Bus Selector8/6 -> [OFDM9_L6_C]  "<L6>"
  Bus Selector8/5 -> [OFDM9_L5_C]  "<L5>"
  Bus Selector8/4 -> [OFDM9_L4_C]  "<L4>"
  Bus Selector8/3 -> [OFDM9_L3_C]  "<L3>"
  Bus Selector8/2 -> [OFDM9_L2_C]  "<L2>"
  Bus Selector8/1 -> [OFDM9_L1_C]  "<L1>"
  Demux16/8 -> [OFDM9_L8]
  Demux16/7 -> [OFDM9_L7]
  Demux16/6 -> [OFDM9_L6]
  Demux16/5 -> [OFDM9_L5]
  Demux16/4 -> [OFDM9_L4]
  Demux16/3 -> [OFDM9_L3]
  Demux16/2 -> [OFDM9_L2]
  Demux16/1 -> [OFDM9_L1]  "OFDM9"
  L_OFDM11/1 -> Demux26/1
  L_OFDM_ctrl11/1 -> Bus Selector10/1
  L_OFDM_ctrl12/1 -> Bus Selector11/1
  L_OFDM12/1 -> Demux28/1
  L_OFDM10/1 -> Demux24/1
  L_OFDM_ctrl10/1 -> Bus Selector9/1
  L_OFDM_ctrl9/1 -> Bus Selector8/1
  L_OFDM9/1 -> Demux16/1
  LAY1/1(TX_L1) -> TX_L1/1
  LAY1/2(TX_valid) -> TX_ctrl1/1
  [OFDM14_L1] -> LAY1/15(L_OFDM14)
  [OFDM13_L1] -> LAY1/16(L_OFDM13)
  [OFDM12_L1] -> LAY1/17(L_OFDM12)
  [OFDM11_L1] -> LAY1/18(L_OFDM11)
  [OFDM10_L1] -> LAY1/19(L_OFDM10)
  [OFDM9_L1] -> LAY1/20(L_OFDM9)
  [OFDM8_L1] -> LAY1/21(L_OFDM8)
  [OFDM7_L1] -> LAY1/22(L_OFDM7)
  [OFDM6_L1] -> LAY1/23(L_OFDM6)
  [OFDM5_L1] -> LAY1/24(L_OFDM5)
  [OFDM4_L1] -> LAY1/25(L_OFDM4)
  [OFDM3_L1] -> LAY1/26(L_OFDM3)
  [OFDM2_L1] -> LAY1/27(L_OFDM2)
  [OFDM1_L1] -> LAY1/28(L_OFDM1)
  [OFDM4_L1_C] -> LAY1/4(L_OFDM_ctrl4)
  [OFDM14_L1_C] -> LAY1/14(L_OFDM_ctrl14)
  [OFDM13_L1_C] -> LAY1/13(L_OFDM_ctrl13)
  [OFDM12_L1_C] -> LAY1/12(L_OFDM_ctrl12)
  [OFDM11_L1_C] -> LAY1/11(L_OFDM_ctrl11)
  [OFDM10_L1_C] -> LAY1/10(L_OFDM_ctrl10)
  [OFDM9_L1_C] -> LAY1/9(L_OFDM_ctrl9)
  [OFDM8_L1_C] -> LAY1/8(L_OFDM_ctrl8)
  [OFDM5_L1_C] -> LAY1/5(L_OFDM_ctrl5)
  [OFDM6_L1_C] -> LAY1/6(L_OFDM_ctrl6)
  [OFDM7_L1_C] -> LAY1/7(L_OFDM_ctrl7)
  [OFDM1_L1_C] -> LAY1/1(L_OFDM_ctrl1)
  [OFDM2_L1_C] -> LAY1/2(L_OFDM_ctrl2)
  [OFDM3_L1_C] -> LAY1/3(L_OFDM_ctrl3)
  [OFDM13_L2] -> LAY2/16(L_OFDM13)
  [OFDM12_L2] -> LAY2/17(L_OFDM12)
  [OFDM11_L2] -> LAY2/18(L_OFDM11)
  [OFDM10_L2] -> LAY2/19(L_OFDM10)
  [OFDM9_L2] -> LAY2/20(L_OFDM9)
  [OFDM8_L2] -> LAY2/21(L_OFDM8)
  [OFDM7_L2] -> LAY2/22(L_OFDM7)
  [OFDM6_L2] -> LAY2/23(L_OFDM6)
  [OFDM5_L2] -> LAY2/24(L_OFDM5)
  [OFDM4_L2] -> LAY2/25(L_OFDM4)
  [OFDM3_L2] -> LAY2/26(L_OFDM3)
  [OFDM2_L2] -> LAY2/27(L_OFDM2)
  [OFDM1_L2] -> LAY2/28(L_OFDM1)
  [OFDM13_L2_C] -> LAY2/13(L_OFDM_ctrl13)
  [OFDM14_L2_C] -> LAY2/14(L_OFDM_ctrl14)
  [OFDM8_L2_C] -> LAY2/8(L_OFDM_ctrl8)
  [OFDM3_L2_C] -> LAY2/3(L_OFDM_ctrl3)
  [OFDM4_L2_C] -> LAY2/4(L_OFDM_ctrl4)
  [OFDM1_L2_C] -> LAY2/1(L_OFDM_ctrl1)
  [OFDM2_L2_C] -> LAY2/2(L_OFDM_ctrl2)
  [OFDM5_L2_C] -> LAY2/5(L_OFDM_ctrl5)
  [OFDM6_L2_C] -> LAY2/6(L_OFDM_ctrl6)
  [OFDM7_L2_C] -> LAY2/7(L_OFDM_ctrl7)
  [OFDM9_L2_C] -> LAY2/9(L_OFDM_ctrl9)
  [OFDM10_L2_C] -> LAY2/10(L_OFDM_ctrl10)
  [OFDM11_L2_C] -> LAY2/11(L_OFDM_ctrl11)
  [OFDM12_L2_C] -> LAY2/12(L_OFDM_ctrl12)
  [OFDM14_L2] -> LAY2/15(L_OFDM14)
  LAY2/1(TX_L1) -> TX_L2/1
  LAY2/2(TX_valid) -> TX_ctrl2/1
  [OFDM14_L3] -> LAY3/15(L_OFDM14)
  [OFDM13_L3] -> LAY3/16(L_OFDM13)
  [OFDM12_L3] -> LAY3/17(L_OFDM12)
  [OFDM11_L3] -> LAY3/18(L_OFDM11)
  [OFDM10_L3] -> LAY3/19(L_OFDM10)
  [OFDM9_L3] -> LAY3/20(L_OFDM9)
  [OFDM8_L3] -> LAY3/21(L_OFDM8)
  [OFDM7_L3] -> LAY3/22(L_OFDM7)
  [OFDM6_L3] -> LAY3/23(L_OFDM6)
  [OFDM5_L3] -> LAY3/24(L_OFDM5)
  [OFDM4_L3] -> LAY3/25(L_OFDM4)
  [OFDM3_L3] -> LAY3/26(L_OFDM3)
  [OFDM2_L3] -> LAY3/27(L_OFDM2)
  [OFDM1_L3] -> LAY3/28(L_OFDM1)
  [OFDM14_L3_C] -> LAY3/14(L_OFDM_ctrl14)
  [OFDM13_L3_C] -> LAY3/13(L_OFDM_ctrl13)
  [OFDM8_L3_C] -> LAY3/8(L_OFDM_ctrl8)
  [OFDM4_L3_C] -> LAY3/4(L_OFDM_ctrl4)
  [OFDM1_L3_C] -> LAY3/1(L_OFDM_ctrl1)
  [OFDM2_L3_C] -> LAY3/2(L_OFDM_ctrl2)
  [OFDM3_L3_C] -> LAY3/3(L_OFDM_ctrl3)
  [OFDM5_L3_C] -> LAY3/5(L_OFDM_ctrl5)
  [OFDM6_L3_C] -> LAY3/6(L_OFDM_ctrl6)
  [OFDM7_L3_C] -> LAY3/7(L_OFDM_ctrl7)
  [OFDM9_L3_C] -> LAY3/9(L_OFDM_ctrl9)
  [OFDM10_L3_C] -> LAY3/10(L_OFDM_ctrl10)
  [OFDM11_L3_C] -> LAY3/11(L_OFDM_ctrl11)
  [OFDM12_L3_C] -> LAY3/12(L_OFDM_ctrl12)
  LAY3/1(TX_L1) -> TX_L3/1
  LAY3/2(TX_valid) -> TX_ctrl3/1
  [OFDM14_L4] -> LAY4/15(L_OFDM14)
  [OFDM13_L4] -> LAY4/16(L_OFDM13)
  [OFDM12_L4] -> LAY4/17(L_OFDM12)
  [OFDM11_L4] -> LAY4/18(L_OFDM11)
  [OFDM10_L4] -> LAY4/19(L_OFDM10)
  [OFDM9_L4] -> LAY4/20(L_OFDM9)
  [OFDM8_L4] -> LAY4/21(L_OFDM8)
  [OFDM7_L4] -> LAY4/22(L_OFDM7)
  [OFDM6_L4] -> LAY4/23(L_OFDM6)
  [OFDM5_L4] -> LAY4/24(L_OFDM5)
  [OFDM4_L4] -> LAY4/25(L_OFDM4)
  [OFDM3_L4] -> LAY4/26(L_OFDM3)
  [OFDM2_L4] -> LAY4/27(L_OFDM2)
  [OFDM1_L4] -> LAY4/28(L_OFDM1)
  [OFDM14_L4_C] -> LAY4/14(L_OFDM_ctrl14)
  [OFDM13_L4_C] -> LAY4/13(L_OFDM_ctrl13)
  [OFDM8_L4_C] -> LAY4/8(L_OFDM_ctrl8)
  [OFDM4_L4_C] -> LAY4/4(L_OFDM_ctrl4)
  [OFDM3_L4_C] -> LAY4/3(L_OFDM_ctrl3)
  [OFDM1_L4_C] -> LAY4/1(L_OFDM_ctrl1)
  [OFDM2_L4_C] -> LAY4/2(L_OFDM_ctrl2)
  [OFDM5_L4_C] -> LAY4/5(L_OFDM_ctrl5)
  [OFDM6_L4_C] -> LAY4/6(L_OFDM_ctrl6)
  [OFDM7_L4_C] -> LAY4/7(L_OFDM_ctrl7)
  [OFDM9_L4_C] -> LAY4/9(L_OFDM_ctrl9)
  [OFDM10_L4_C] -> LAY4/10(L_OFDM_ctrl10)
  [OFDM11_L4_C] -> LAY4/11(L_OFDM_ctrl11)
  [OFDM12_L4_C] -> LAY4/12(L_OFDM_ctrl12)
  LAY4/1(TX_L1) -> TX_L4/1
  LAY4/2(TX_valid) -> TX_ctrl4/1
  [OFDM14_L5] -> LAY9/15(L_OFDM14)
  [OFDM13_L5] -> LAY9/16(L_OFDM13)
  [OFDM12_L5] -> LAY9/17(L_OFDM12)
  [OFDM11_L5] -> LAY9/18(L_OFDM11)
  [OFDM10_L5] -> LAY9/19(L_OFDM10)
  [OFDM9_L5] -> LAY9/20(L_OFDM9)
  [OFDM8_L5] -> LAY9/21(L_OFDM8)
  [OFDM7_L5] -> LAY9/22(L_OFDM7)
  [OFDM6_L5] -> LAY9/23(L_OFDM6)
  [OFDM5_L5] -> LAY9/24(L_OFDM5)
  [OFDM4_L5] -> LAY9/25(L_OFDM4)
  [OFDM3_L5] -> LAY9/26(L_OFDM3)
  [OFDM2_L5] -> LAY9/27(L_OFDM2)
  [OFDM1_L5] -> LAY9/28(L_OFDM1)
  [OFDM4_L5_C] -> LAY9/4(L_OFDM_ctrl4)
  [OFDM3_L5_C] -> LAY9/3(L_OFDM_ctrl3)
  [OFDM2_L5_C] -> LAY9/2(L_OFDM_ctrl2)
  [OFDM1_L5_C] -> LAY9/1(L_OFDM_ctrl1)
  [OFDM5_L5_C] -> LAY9/5(L_OFDM_ctrl5)
  [OFDM6_L5_C] -> LAY9/6(L_OFDM_ctrl6)
  [OFDM7_L5_C] -> LAY9/7(L_OFDM_ctrl7)
  [OFDM8_L5_C] -> LAY9/8(L_OFDM_ctrl8)
  [OFDM9_L5_C] -> LAY9/9(L_OFDM_ctrl9)
  [OFDM10_L5_C] -> LAY9/10(L_OFDM_ctrl10)
  [OFDM11_L5_C] -> LAY9/11(L_OFDM_ctrl11)
  [OFDM12_L5_C] -> LAY9/12(L_OFDM_ctrl12)
  [OFDM13_L5_C] -> LAY9/13(L_OFDM_ctrl13)
  [OFDM14_L5_C] -> LAY9/14(L_OFDM_ctrl14)
  LAY9/1(TX_L1) -> TX_L5/1
  LAY9/2(TX_valid) -> TX_ctrl5/1
  [OFDM14_L6] -> LAY5/15(L_OFDM14)
  [OFDM13_L6] -> LAY5/16(L_OFDM13)
  [OFDM12_L6] -> LAY5/17(L_OFDM12)
  [OFDM11_L6] -> LAY5/18(L_OFDM11)
  [OFDM10_L6] -> LAY5/19(L_OFDM10)
  [OFDM9_L6] -> LAY5/20(L_OFDM9)
  [OFDM8_L6] -> LAY5/21(L_OFDM8)
  [OFDM7_L6] -> LAY5/22(L_OFDM7)
  [OFDM6_L6] -> LAY5/23(L_OFDM6)
  [OFDM5_L6] -> LAY5/24(L_OFDM5)
  [OFDM4_L6] -> LAY5/25(L_OFDM4)
  [OFDM3_L6] -> LAY5/26(L_OFDM3)
  [OFDM2_L6] -> LAY5/27(L_OFDM2)
  [OFDM1_L6] -> LAY5/28(L_OFDM1)
  [OFDM14_L6_C] -> LAY5/14(L_OFDM_ctrl14)
  [OFDM13_L6_C] -> LAY5/13(L_OFDM_ctrl13)
  [OFDM9_L6_C] -> LAY5/9(L_OFDM_ctrl9)
  [OFDM10_L6_C] -> LAY5/10(L_OFDM_ctrl10)
  [OFDM11_L6_C] -> LAY5/11(L_OFDM_ctrl11)
  [OFDM12_L6_C] -> LAY5/12(L_OFDM_ctrl12)
  [OFDM8_L6_C] -> LAY5/8(L_OFDM_ctrl8)
  [OFDM7_L6_C] -> LAY5/7(L_OFDM_ctrl7)
  [OFDM5_L6_C] -> LAY5/5(L_OFDM_ctrl5)
  [OFDM6_L6_C] -> LAY5/6(L_OFDM_ctrl6)
  [OFDM4_L6_C] -> LAY5/4(L_OFDM_ctrl4)
  [OFDM3_L6_C] -> LAY5/3(L_OFDM_ctrl3)
  [OFDM1_L6_C] -> LAY5/1(L_OFDM_ctrl1)
  [OFDM2_L6_C] -> LAY5/2(L_OFDM_ctrl2)
  LAY5/1(TX_L1) -> TX_L6/1
  LAY5/2(TX_valid) -> TX_ctrl6/1
  [OFDM14_L7] -> LAY6/15(L_OFDM14)
  [OFDM13_L7] -> LAY6/16(L_OFDM13)
  [OFDM12_L7] -> LAY6/17(L_OFDM12)
  [OFDM11_L7] -> LAY6/18(L_OFDM11)
  [OFDM10_L7] -> LAY6/19(L_OFDM10)
  [OFDM9_L7] -> LAY6/20(L_OFDM9)
  [OFDM8_L7] -> LAY6/21(L_OFDM8)
  [OFDM7_L7] -> LAY6/22(L_OFDM7)
  [OFDM6_L7] -> LAY6/23(L_OFDM6)
  [OFDM5_L7] -> LAY6/24(L_OFDM5)
  [OFDM4_L7] -> LAY6/25(L_OFDM4)
  [OFDM3_L7] -> LAY6/26(L_OFDM3)
  [OFDM2_L7] -> LAY6/27(L_OFDM2)
  [OFDM1_L7] -> LAY6/28(L_OFDM1)
  [OFDM14_L7_C] -> LAY6/14(L_OFDM_ctrl14)
  [OFDM13_L7_C] -> LAY6/13(L_OFDM_ctrl13)
  [OFDM5_L7_C] -> LAY6/5(L_OFDM_ctrl5)
  [OFDM6_L7_C] -> LAY6/6(L_OFDM_ctrl6)
  [OFDM7_L7_C] -> LAY6/7(L_OFDM_ctrl7)
  [OFDM8_L7_C] -> LAY6/8(L_OFDM_ctrl8)
  [OFDM9_L7_C] -> LAY6/9(L_OFDM_ctrl9)
  [OFDM10_L7_C] -> LAY6/10(L_OFDM_ctrl10)
  [OFDM11_L7_C] -> LAY6/11(L_OFDM_ctrl11)
  [OFDM12_L7_C] -> LAY6/12(L_OFDM_ctrl12)
  [OFDM4_L7_C] -> LAY6/4(L_OFDM_ctrl4)
  [OFDM3_L7_C] -> LAY6/3(L_OFDM_ctrl3)
  [OFDM1_L7_C] -> LAY6/1(L_OFDM_ctrl1)
  [OFDM2_L7_C] -> LAY6/2(L_OFDM_ctrl2)
  LAY6/1(TX_L1) -> TX_L7/1
  LAY6/2(TX_valid) -> TX_ctrl7/1
  [OFDM14_L8] -> LAY7/15(L_OFDM14)
  [OFDM13_L8] -> LAY7/16(L_OFDM13)
  [OFDM12_L8] -> LAY7/17(L_OFDM12)
  [OFDM11_L8] -> LAY7/18(L_OFDM11)
  [OFDM10_L8] -> LAY7/19(L_OFDM10)
  [OFDM9_L8] -> LAY7/20(L_OFDM9)
  [OFDM8_L8] -> LAY7/21(L_OFDM8)
  [OFDM7_L8] -> LAY7/22(L_OFDM7)
  [OFDM6_L8] -> LAY7/23(L_OFDM6)
  [OFDM5_L8] -> LAY7/24(L_OFDM5)
  [OFDM4_L8] -> LAY7/25(L_OFDM4)
  [OFDM3_L8] -> LAY7/26(L_OFDM3)
  [OFDM2_L8] -> LAY7/27(L_OFDM2)
  [OFDM1_L8] -> LAY7/28(L_OFDM1)
  [OFDM14_L8_C] -> LAY7/14(L_OFDM_ctrl14)
  [OFDM13_L8_C] -> LAY7/13(L_OFDM_ctrl13)
  [OFDM9_L8_C] -> LAY7/9(L_OFDM_ctrl9)
  [OFDM10_L8_C] -> LAY7/10(L_OFDM_ctrl10)
  [OFDM11_L8_C] -> LAY7/11(L_OFDM_ctrl11)
  [OFDM12_L8_C] -> LAY7/12(L_OFDM_ctrl12)
  [OFDM5_L8_C] -> LAY7/5(L_OFDM_ctrl5)
  [OFDM6_L8_C] -> LAY7/6(L_OFDM_ctrl6)
  [OFDM7_L8_C] -> LAY7/7(L_OFDM_ctrl7)
  [OFDM8_L8_C] -> LAY7/8(L_OFDM_ctrl8)
  [OFDM4_L8_C] -> LAY7/4(L_OFDM_ctrl4)
  [OFDM3_L8_C] -> LAY7/3(L_OFDM_ctrl3)
  [OFDM2_L8_C] -> LAY7/2(L_OFDM_ctrl2)
  [OFDM1_L8_C] -> LAY7/1(L_OFDM_ctrl1)
  LAY7/1(TX_L1) -> TX_L8/1
  LAY7/2(TX_valid) -> TX_ctrl8/1

== system tx2/NR DL process0 ==
  ctrl_process2 : Inport
  Bus Creator : BusCreator  Inputs=8  OutDataTypeStr=Bus: BUSOFDM1
  Delay : Delay  DelayLength=1  InitialCondition=0
  Delay1 : Delay  InitialCondition=0
  Delay2 : Delay  InitialCondition=0
  Delay3 : Delay  InitialCondition=0
  Delay4 : Delay  DelayLength=1  InitialCondition=0
  Delay5 : Delay  DelayLength=1  InitialCondition=0
  Detect Fall Nonpositive : hdlsllib/Logic and Bit Operations/Detect Fall Nonpositive  vinit=0  OutDataTypeStr=boolean
      settings: SourceProductBaseCode=SL
  Ground : Ground
  HDL Counter : hdlsllib/Sources/HDL Counter  CountType=Count limited  CountInit=0  CountStep=1  CountMax=1159  CountFromType=Initial value  CountFrom=0  CountResetPort=on  CountLoadPort=off  CountEnbPort=on  CountDirPort=off  CountHitOutputPort=off  CountDataType=Unsigned  CountWordLen=16  CountFracLen=0  CountSampTime=1
  Logical Operator : Logic  AllPortsSameDT=off  OutDataTypeStr=boolean
  Logical Operator1 : Logic  Operator=NOT  AllPortsSameDT=off  OutDataTypeStr=boolean
  Mux : Mux  Inputs=8
  Sample Control Bus Creator : whdlutilities/Sample Control Bus Creator
      settings: SourceProductBaseCode=LH
  Sample Control Bus Selector : whdlutilities/Sample Control Bus Selector  OutputSignals=start,end,valid
      settings: SourceProductBaseCode=LH
  Subsystem1 : Subsystem  mask{valid_length=4548}
      mask prompts: valid_length "The length of valid"
      mask DialogControl Control2 Prompt: Latency=2
  Subsystem2 : Subsystem  mask{valid_length=1160}
      mask prompts: valid_length "The length of valid"
      mask DialogControl Control2 Prompt: Latency=2
  Switch : Switch  Criteria=u2 ~= 0  SaturateOnIntegerOverflow=off  InputSameDT=off
  Terminator : Terminator
  Terminator1 : Terminator
  rom_bf2 : Subsystem
  L_OFDM1 : Outport
  L_OFDM_ctrl1 : Outport  Port=2  OutDataTypeStr=Bus: BUSOFDM1
  wires:
  Sample Control Bus Creator/1 -> Bus Creator/8, Bus Creator/7, Bus Creator/6, Bus Creator/5, Bus Creator/4, Bus Creator/3, Bus Creator/2, Bus Creator/1  "rom_valid"
  Subsystem2/1(valid_out) -> Delay1/1, HDL Counter/2, Logical Operator1/1  "valid_out"
  Sample Control Bus Selector/2 -> Terminator1/1  "<end>"
  Delay/1 -> Logical Operator/1
  Subsystem2/3(end_out) -> Delay3/1  "end"
  ctrl_process2/1 -> Sample Control Bus Selector/1
  Switch/1 -> Mux/7, Mux/8, Mux/6, Mux/5, Mux/4, Mux/1, Mux/2, Mux/3  "rom_data"
  Sample Control Bus Selector/1 -> Subsystem1/1(start)  "<start>"
  Subsystem1/1(valid_out) -> Detect Fall Nonpositive/1, Delay/1  "count"
  Logical Operator/1 -> Subsystem2/1(start)
  Detect Fall Nonpositive/1 -> Logical Operator/2
  HDL Counter/1 -> rom_bf2/1(address)
  Logical Operator1/1 -> HDL Counter/1
  Subsystem2/2(start_out) -> Delay2/1
  Mux/1 -> Delay4/1
  Sample Control Bus Selector/3 -> Terminator/1  "<valid>"
  Delay1/1 -> Sample Control Bus Creator/3, Switch/2  "rom_valid"
  Delay2/1 -> Sample Control Bus Creator/1  "rom_start"
  Delay3/1 -> Sample Control Bus Creator/2  "rom_end"
  rom_bf2/1(data_out) -> Switch/1  "rom_data"
  Ground/1 -> Switch/3
  Delay4/1 -> L_OFDM1/1
  Bus Creator/1 -> Delay5/1
  Delay5/1 -> L_OFDM_ctrl1/1
